simulink model "tpt"  (Simulink 6.6)
settings: Solver=ode45  StartTime=0.0  StopTime=10.0  RelTol=1e-3
libraries: cdsFilt x154, cdsMatrix x16, cdsEpicsIn x13, cdsEpicsOut x11, cdsOsc x5, cdsPhase x5, dac x1, simulink x1, cdsParameters x1
(part 1 of 8)
settings Model: Creator=jay  LastModifiedBy=controls  ExtModeAutoUpdateStatusClock=off
settings DebuggingCC: SignalResolutionControl=TryResolveAllWithWarning  MultiTaskDSMMsg=warning  MultiTaskCondExecSysMsg=none  StrictBusMsg=None
settings RTWCC: IncludeERTFirstTime=on

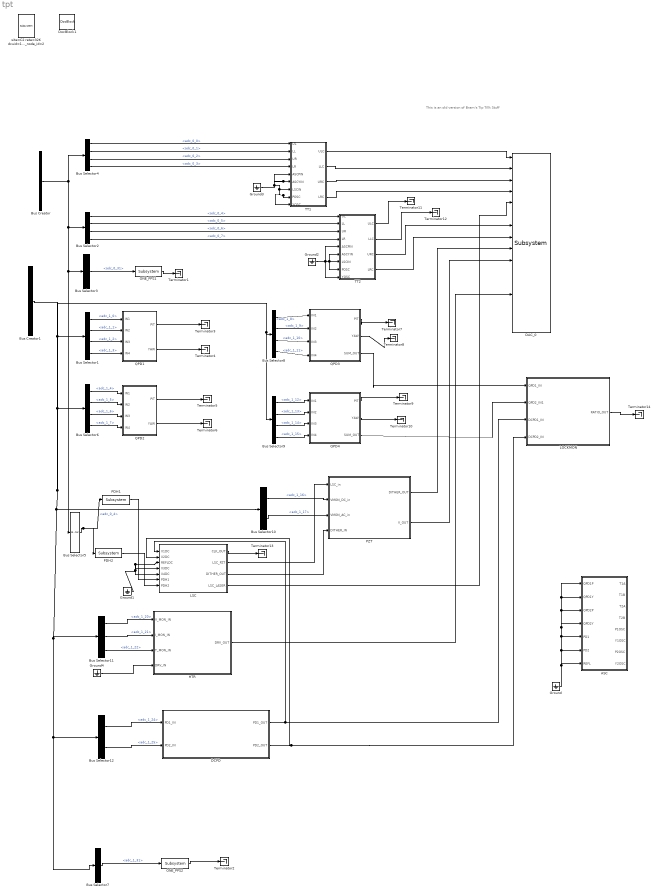
== system tpt ==
  note: This is an old version of Bram's Tip Tillt Stuff
  ASC : Subsystem
  Bus Creator : BusCreator  Tag=adc_0  Description=|  Inputs='adc_0_0','adc_0_1','adc_0_2','adc_0_3','adc_0_4','adc_0_5','adc_0_6','adc_0_7','adc_0_8','adc_0_9','adc_0_10','adc_0_11','adc_0_12','adc_0_13','adc_0_14','adc_0_15','adc_0_16','adc_0_17','adc_0_18','adc_0_19','adc_0_20','adc_0_21','adc_0_22','adc_0_23','adc_0_24','adc_0_25','adc_0_26','adc_0_27','adc_0_28','adc_0_29','adc_0_30','adc_0_31'
      | PCI66-16AI64SSA
      | 40Vp-p, 16-bit, 610uV/count
      settings: AttributesFormatString=%<Description>\n%<Tag>
  Bus Creator1 : BusCreator  Tag=adc_1  Description=|  Inputs='adc_1_0','adc_1_1','adc_1_2','adc_1_3','adc_1_4','adc_1_5','adc_1_6','adc_1_7','adc_1_8','adc_1_9','adc_1_10','adc_1_11','adc_1_12','adc_1_13','adc_1_14','adc_1_15','adc_1_16','adc_1_17','adc_1_18','adc_1_19','adc_1_20','adc_1_21','adc_1_22','adc_1_23','adc_1_24','adc_1_25','adc_1_26','adc_1_27','adc_1_28','adc_1_29','adc_1_30','adc_1_31'
      | PCI66-16AI64SSA
      | 40Vp-p, 16-bit, 610uV/count
      settings: AttributesFormatString=%<Description>\n%<Tag>
  Bus Selector1 : BusSelector  OutputSignals=adc_1_0,adc_1_1,adc_1_2,adc_1_3
  Bus Selector10 : BusSelector  OutputSignals=adc_1_16,adc_1_17
  Bus Selector11 : BusSelector  OutputSignals=adc_1_20,adc_1_21,adc_1_22
  Bus Selector12 : BusSelector  OutputSignals=adc_1_24,adc_1_25
  Bus Selector2 : BusSelector  OutputSignals=adc_0_4,adc_0_5,adc_0_6,adc_0_7
  Bus Selector3 : BusSelector  OutputSignals=adc_0_31
  Bus Selector4 : BusSelector  OutputSignals=adc_0_0,adc_0_1,adc_0_2,adc_0_3
  Bus Selector5 : BusSelector  OutputSignals=adc_0_4
  Bus Selector6 : BusSelector  OutputSignals=adc_1_4,adc_1_5,adc_1_6,adc_1_7
  Bus Selector7 : BusSelector  OutputSignals=adc_1_31
  Bus Selector8 : BusSelector  OutputSignals=adc_1_8,adc_1_9,adc_1_10,adc_1_11
  Bus Selector9 : BusSelector  OutputSignals=adc_1_12,adc_1_13,adc_1_14,adc_1_15
  DAC_0 : dac/Subsystem  Description=|  SystemSampleTime=-1
      | PCI66-16AO16
      | 20Vp-p, 16-bit, 305uV/count
      settings: AttributesFormatString=%<Description>
  DCPD : Subsystem
  DocBlock1 : simulink/Model-Wide Utilities/DocBlock  Tag=SW Install  SystemSampleTime=-1  DocumentType=Text
      content=|
      | *******************************************************
      | Software installation on new computer
      | *******************************************************
      |
      | 1. Install network and PCIe cards.
      |     - Remove top cover and I/O cage.
      |     - Install NIC in PCI-X slot.
      |     - Install PCIe card for I/O chassis in PCIe slot.
      |     - Reinstall I/O cage.
      |     - Close cover.
      | 2. Connect Infiniband cables to I/O chassis and power up I/O chassis.
      | 3. Power up computer.
      | 4. Change root password.
      | 5. Modify network startup.
      |     - edit /etc/sysconfig/network-scripts (can remove all except eth0)
      |     - Change hostname in /etc/sysconfig/network file
      |     - Modify /etc/hosts
      | 6. Add users
      | 7. Make rtLinux
      |     - cd to kernel directory
      |     - Type 'make modules-install install
      |     - Edit /etc/grub_conf and change default to 0 to boot rtLinux on powerup.
      | 8. Get rid of unnecessary tasks.
      |     - cpuspeed
      |     - bluetooth
      |     - avahi daemon
      |     - cups
      |     - cups config
      |     - httpd
      |     - haldaemon
      |     - hidd
      |     - iptables
      |     - isdn
      |     - kudsu
      |     - sendmail
      |     - smartd
      |     - xfs
      | 9. reboot
      | 10. Use del key to bring up boot configuration and get rid of all unnecessary support, such as:
      |     - parallel, serial ports
      |     - USB
      | 11. Install CDS EPICS files
      |     - cd to /opt
      |     - load CDS CD (mount /dev/cdrom /mnt)
      |     - Run 'tar zxf /mnt/epics.tar.gz'
      | 12. Edit /etc/rc.local file and add:
      |     - /opt/rtlinux_dir/rtlinuxpro/mdoules/rtcore&
      |     - /opt/epics-3.14.7-linux/base/bin/linux-x86/caRepeater&
      |     - sleep 5
      |     - /etc/setup_shmem.rtl&
      | 13. Add EPICS libraries to all paths
      |     - cd to /etc/ld.so.conf.d
      |     - edit epics.conf
      |     - Add the following lines to this file:
      |         - /opt/epics-3.14.7-linux/base/lib/linux-x86
      |         - /opt/epics-3.14.7-linux/seq/lib/linux-x86
      | 14. Add CDS source code.
      |     - cd to /home/user
      |     - tar zxf /mnt/cds.tar.gz
      | 15. Build the shmem module.
      |     - cd to /home/user/cds/advLigo/src/fe/shmem
      |     - Type 'make'
      |     - cp shmem.rtl file to /etc
      | 16. Run the rc local file.
      |     - /etc/rc.local
      | 17. Create the gm files.
      |     - untar gm files in root home directory.
      |     - Type make.
      |     - Go to gm binary directory.
      |     - mkdir /opt/gm
      |     - ./GM_INSTALL
      |     - chkconfig --add gm
      |     - chkconfig gm on
      |     - service gm start
      | 18. Need to get rid of possible errors in running sequences looking for caRepeater.
      |     - ln -s /bin/true /bin/caRepeater
      | 19. Reboot
      |
      | ******* Should now be able to build FE code and EPICS.
      settings: AttributesFormatString=%<Tag>
  Ground{,1..4} (5 alike) : Ground
  HTR : Subsystem
  LOCKMON : Subsystem
  LSC : Subsystem
  ONE_PPS1 : cdsFilt/Subsystem  Tag=cdsFilt  Description=|  SystemSampleTime=-1
      | Purpose:                                                                                                                                                                                                                                  
      | Standard CDS IIR filter module.                                                                                                                                                                                                           
      |                                                                                                                                                                                                                                           
      | Operation:                                                                                                                                                                                                                                
      | Consists of 10 second order section IIR filters, plus a ramped gain stage. In FE code, also provides pre-defined test points and excitation channel inputs. The filter coefficients are defined in the LIGO system using the 'foton' tool.
      |                                                                                                                                                                                                                                           
      | Usage:                                                                                                                                                                                                                                    
      | Name the part with the desired filter module name.
      settings: AttributesFormatString=%<Tag>
  ONE_PPS2 : cdsFilt/Subsystem  Tag=cdsFilt  Description=|  SystemSampleTime=-1
      | Purpose:                                                                                                                                                                                                                                  
      | Standard CDS IIR filter module.                                                                                                                                                                                                           
      |                                                                                                                                                                                                                                           
      | Operation:                                                                                                                                                                                                                                
      | Consists of 10 second order section IIR filters, plus a ramped gain stage. In FE code, also provides pre-defined test points and excitation channel inputs. The filter coefficients are defined in the LIGO system using the 'foton' tool.
      |                                                                                                                                                                                                                                           
      | Usage:                                                                                                                                                                                                                                    
      | Name the part with the desired filter module name.
      settings: AttributesFormatString=%<Tag>
  PDH1 : cdsFilt/Subsystem  Tag=cdsFilt  Description=|  SystemSampleTime=-1
      | Purpose:                                                                                                                                                                                                                                  
      | Standard CDS IIR filter module.                                                                                                                                                                                                           
      |                                                                                                                                                                                                                                           
      | Operation:                                                                                                                                                                                                                                
      | Consists of 10 second order section IIR filters, plus a ramped gain stage. In FE code, also provides pre-defined test points and excitation channel inputs. The filter coefficients are defined in the LIGO system using the 'foton' tool.
      |                                                                                                                                                                                                                                           
      | Usage:                                                                                                                                                                                                                                    
      | Name the part with the desired filter module name.
      link override Digital Filter0: NumCoeffs=[1]  DenCoeffs=[1]
      settings: AttributesFormatString=%<Tag>
  PDH2 : cdsFilt/Subsystem  Tag=cdsFilt  Description=|  SystemSampleTime=-1
      | Purpose:                                                                                                                                                                                                                                  
      | Standard CDS IIR filter module.                                                                                                                                                                                                           
      |                                                                                                                                                                                                                                           
      | Operation:                                                                                                                                                                                                                                
      | Consists of 10 second order section IIR filters, plus a ramped gain stage. In FE code, also provides pre-defined test points and excitation channel inputs. The filter coefficients are defined in the LIGO system using the 'foton' tool.
      |                                                                                                                                                                                                                                           
      | Usage:                                                                                                                                                                                                                                    
      | Name the part with the desired filter module name.
      settings: AttributesFormatString=%<Tag>
  PZT : Subsystem
  QPD1 : Subsystem  Description=QPD Monitors of Table-- SUM, PIT, YAW
      settings: AttributesFormatString=%<Description>
  QPD2 : Subsystem  Description=QPD Monitors of Table-- SUM, PIT, YAW
      settings: AttributesFormatString=%<Description>
  QPD3 : Subsystem  Description=QPD Monitors of Table-- SUM, PIT, YAW
      settings: AttributesFormatString=%<Description>
  QPD4 : Subsystem  Description=QPD Monitors of Table-- SUM, PIT, YAW
      settings: AttributesFormatString=%<Description>
  TT1 : Subsystem
  TT2 : Subsystem
  Terminator{1..14} (14 alike) : Terminator
  site=C2 rate=32K dcuid=10 gds_node_id=2 : cdsParameters/Subsystem  Tag=cdsParameters  SystemSampleTime=-1
      settings: AttributesFormatString=%<Tag>
  wires:
  Bus Creator/1 -> Bus Selector4/1, Bus Selector2/1, Bus Selector3/1, Bus Selector5/1
  Bus Selector4/1 -> TT1/1(UL)  "<adc_0_0>"
  Bus Selector4/2 -> TT1/2(LL)  "<adc_0_1>"
  Bus Selector4/3 -> TT1/3(UR)  "<adc_0_2>"
  Bus Selector4/4 -> TT1/4(LR)  "<adc_0_3>"
  TT1/1(ULC) -> DAC_0/1
  TT1/2(LLC) -> DAC_0/2
  TT1/3(URC) -> DAC_0/3
  TT1/4(LRC) -> DAC_0/4
  Bus Selector2/4 -> TT2/4(LR)  "<adc_0_7>"
  Bus Selector2/1 -> TT2/1(UL)  "<adc_0_4>"
  Bus Selector2/2 -> TT2/2(LL)  "<adc_0_5>"
  Bus Selector2/3 -> TT2/3(UR)  "<adc_0_6>"
  TT2/4(LRC) -> DAC_0/8
  TT2/3(URC) -> DAC_0/7
  Ground2/1 -> TT2/5(ASCPIN), TT2/9(YOSC), TT2/7(LSCIN), TT2/6(ASCYIN), TT2/8(POSC)
  ONE_PPS1/1 -> Terminator1/1
  Bus Selector3/1 -> ONE_PPS1/1  "<adc_0_31>"
  Bus Selector1/1 -> QPD1/1(IN1)  "<adc_1_0>"
  Bus Selector1/2 -> QPD1/2(IN2)  "<adc_1_1>"
  Bus Selector1/3 -> QPD1/3(IN3)  "<adc_1_2>"
  Bus Selector1/4 -> QPD1/4(IN4)  "<adc_1_3>"
  Bus Selector5/1 -> PDH1/1, PDH2/1  "<adc_0_4>"
  Bus Selector6/1 -> QPD2/1(IN1)  "<adc_1_4>"
  Bus Selector6/2 -> QPD2/2(IN2)  "<adc_1_5>"
  Bus Selector6/3 -> QPD2/3(IN3)  "<adc_1_6>"
  Bus Selector6/4 -> QPD2/4(IN4)  "<adc_1_7>"
  Bus Creator1/1 -> Bus Selector1/1, Bus Selector6/1, Bus Selector8/1, Bus Selector9/1, Bus Selector10/1, Bus Selector11/1, Bus Selector7/1, Bus Selector12/1
  ONE_PPS2/1 -> Terminator2/1
  Bus Selector7/1 -> ONE_PPS2/1  "<adc_1_31>"
  Ground3/1 -> TT1/5(ASCPIN), TT1/6(ASCYIN), TT1/8(POSC), TT1/9(YOSC), TT1/7(LSCIN)
  QPD1/2(YAW) -> Terminator4/1
  QPD1/1(PIT) -> Terminator3/1
  QPD2/2(YAW) -> Terminator6/1
  QPD2/1(PIT) -> Terminator5/1
  Bus Selector8/1 -> QPD3/1(IN1)  "<adc_1_8>"
  Bus Selector8/2 -> QPD3/2(IN2)  "<adc_1_9>"
  Bus Selector8/3 -> QPD3/3(IN3)  "<adc_1_10>"
  Bus Selector8/4 -> QPD3/4(IN4)  "<adc_1_11>"
  QPD3/2(YAW) -> Terminator8/1
  QPD3/1(PIT) -> Terminator7/1
  Bus Selector9/1 -> QPD4/1(IN1)  "<adc_1_12>"
  Bus Selector9/2 -> QPD4/2(IN2)  "<adc_1_13>"
  Bus Selector9/3 -> QPD4/3(IN3)  "<adc_1_14>"
  Bus Selector9/4 -> QPD4/4(IN4)  "<adc_1_15>"
  QPD4/1(PIT) -> Terminator9/1
  PDH1/1 -> LSC/6(PDH1)
  Bus Selector10/1 -> PZT/2(VMON_DC_in)  "<adc_1_16>"
  Bus Selector10/2 -> PZT/3(VMON_AC_in)  "<adc_1_17>"
  PZT/1(DITHER_OUT) -> DAC_0/9
  PZT/2(V_OUT) -> DAC_0/10
  TT2/1(ULC) -> Terminator11/1
  TT2/2(LLC) -> Terminator12/1
  Ground/1 -> ASC/4(QPD2Y), ASC/1(QPD1P), ASC/2(QPD1Y), ASC/3(QPD2P), ASC/5(PD1), ASC/6(PD2), ASC/7(REFL)
  Ground1/1 -> LSC/5(X4DC), LSC/4(X3DC), LSC/3(REFLDC)
  LSC/1(CLK_OUT) -> Terminator13/1
  LSC/3(DITHER_OUT) -> PZT/4(DITHER_IN)
  Bus Selector11/1 -> HTR/1(V_MON_IN)  "<adc_1_20>"
  Bus Selector11/2 -> HTR/2(I_MON_IN)  "<adc_1_21>"
  Bus Selector11/3 -> HTR/3(T_MON_IN)  "<adc_1_22>"
  Ground4/1 -> HTR/4(DRV_IN)
  HTR/1(DRV_OUT) -> DAC_0/13
  Bus Selector12/1 -> DCPD/1(PD1_IN)  "<adc_1_24>"
  Bus Selector12/2 -> DCPD/2(PD2_IN)  "<adc_1_25>"
  PDH2/1 -> LSC/7(PDH2)
  QPD4/2(YAW) -> Terminator10/1
  QPD3/3(SUM_OUT) -> LOCKMON/1(QPD1_IN)
  QPD4/3(SUM_OUT) -> LOCKMON/2(QPD2_IN1)
  DCPD/1(PD1_OUT) -> LOCKMON/3(DCPD1_IN), LSC/1(X1DC)
  DCPD/2(PD2_OUT) -> LSC/2(X2DC), LOCKMON/4(DCPD2_IN)
  LOCKMON/1(RATIO_OUT) -> Terminator14/1
  LSC/2(LSC_PZT) -> PZT/1(LSC_in)
  LSC/4(LSC_LASER) -> DAC_0/5
